simulink model "Scenario_1"  (R2020b)
settings: Solver=ode1  StartTime=0.0  StopTime=10  FixedStep=Ts  RelTol=1e-3
InitFcn:
  | Scenario_1_parameters;
values from neighbouring files (symbols this model uses):
  c0 = c0_zeb    (= 6.57988e-09)    [Scenario_17_parameters.m]    (also in Scenario_1_parameters.m = 6.37282e-09; Scenario_2_parameters.m = 6.37282e-09; Scenario_3_parameters.m)
  c1 = c1_zeb    (= 9.15905e-09)    [Scenario_17_parameters.m]    (also in Scenario_1_parameters.m = 8.76156e-09; Scenario_2_parameters.m = 8.76156e-09; Scenario_3_parameters.m)
  fg = 50    [Scenario_17_parameters.m]    (also in Scenario_1_parameters.m; Scenario_2_parameters.m; Scenario_3_parameters.m)
  G1gen = 0.50    (= 0.5)    [Scenario_17_parameters.m]    (also in Scenario_1_parameters.m = 0.2; Scenario_2_parameters.m = 0.1245; Scenario_3_parameters.m = 0.45)
  G2gen = 0.30    (= 0.3)    [Scenario_1_parameters.m]    (also in Scenario_2_parameters.m; Scenario_3_parameters.m = 0.4)
  G3gen = 0.25    [Scenario_1_parameters.m]    (also in Scenario_2_parameters.m = 0.2; Scenario_3_parameters.m = 0.6)
  G5gen = 0.75    [Scenario_17_parameters.m]    (also in Scenario_1_parameters.m = 0.22; Scenario_2_parameters.m = 0.2; Scenario_3_parameters.m = 0.7)
  G6gen = 0.90    (= 0.9)    [Scenario_17_parameters.m]    (also in Scenario_1_parameters.m = 0.41; Scenario_2_parameters.m = 0.2078; Scenario_3_parameters.m = 0.95)
  G7gen = 0.60    (= 0.6)    [Scenario_17_parameters.m]    (also in Scenario_1_parameters.m = 0.52; Scenario_2_parameters.m = 0.518; Scenario_3_parameters.m = 0.5)
  Ihvpk = Ihv*sqrt(2)    [Scenario_17_parameters.m]    (also in Scenario_1_parameters.m; Scenario_2_parameters.m; Scenario_3_parameters.m)
  l0 = l0_zeb    (= 0.00368)    [Scenario_17_parameters.m]    (also in Scenario_1_parameters.m = 0.00373; Scenario_2_parameters.m = 0.00373; Scenario_3_parameters.m)
  l1 = l1_zeb    (= 0.00128)    [Scenario_17_parameters.m]    (also in Scenario_1_parameters.m = 0.00133; Scenario_2_parameters.m = 0.00133; Scenario_3_parameters.m)
  L3dem = 0.30    (= 0.3)    [Scenario_17_parameters.m]    (also in Scenario_1_parameters.m = 0.1; Scenario_2_parameters.m = 0.1; Scenario_3_parameters.m = 0.2)
  L4dem = 0.30    (= 0.3)    [Scenario_1_parameters.m]    (also in Scenario_2_parameters.m)
  L5dem = 0.25    [Scenario_17_parameters.m]    (also in Scenario_1_parameters.m = 0.35; Scenario_2_parameters.m = 0.35)
  L6dem = 0.15    [Scenario_1_parameters.m]    (also in Scenario_2_parameters.m; Scenario_3_parameters.m = 0.1)
  L7dem = 0.10    (= 0.1)    [Scenario_1_parameters.m]    (also in Scenario_2_parameters.m; Scenario_3_parameters.m = 0.15)
  Pr = Sr*PF    (= 1900000000)    [Scenario_17_parameters.m]    (also in Scenario_1_parameters.m = 550050000; Scenario_2_parameters.m = 550050000; Scenario_3_parameters.m = 11640000000)
  Qr = sqrt(Sr^2 - Pr^2)    [Scenario_17_parameters.m]    (also in Scenario_1_parameters.m; Scenario_2_parameters.m; Scenario_3_parameters.m)
  r0 = r0_zeb    (= 0.39362)    [Scenario_17_parameters.m]    (also in Scenario_1_parameters.m = 0.44587; Scenario_2_parameters.m = 0.44587; Scenario_3_parameters.m)
  r1 = r1_zeb    (= 0.06862)    [Scenario_17_parameters.m]    (also in Scenario_1_parameters.m = 0.12087; Scenario_2_parameters.m = 0.12087; Scenario_3_parameters.m)
  Rtpu = Xtpu/40    (= 0.0025)    [Scenario_17_parameters.m]    (also in Scenario_1_parameters.m = 0.00375; Scenario_2_parameters.m = 0.00375; Scenario_3_parameters.m = 0.00375)
  S1non = 700e6    (= 700000000)    [Scenario_17_parameters.m]    (also in Scenario_1_parameters.m = 400000000; Scenario_2_parameters.m = 400000000; Scenario_3_parameters.m = 1000000000)
  S2non = 300e6    (= 300000000)    [Scenario_1_parameters.m]    (also in Scenario_2_parameters.m; Scenario_3_parameters.m = 3000000000)
  S3non = 200e6    (= 200000000)    [Scenario_1_parameters.m]    (also in Scenario_2_parameters.m; Scenario_3_parameters.m = 1000000000)
  S5non = 400e6    (= 400000000)    [Scenario_17_parameters.m]    (also in Scenario_1_parameters.m = 500000000; Scenario_2_parameters.m = 500000000; Scenario_3_parameters.m = 2000000000)
  S6non = 150e6    (= 150000000)    [Scenario_17_parameters.m]    (also in Scenario_1_parameters.m = 400000000; Scenario_2_parameters.m = 400000000; Scenario_3_parameters.m = 3000000000)
  S7non = 1000e6    (= 1000000000)    [Scenario_17_parameters.m]    (also in Scenario_1_parameters.m = 200000000; Scenario_2_parameters.m = 200000000; Scenario_3_parameters.m = 4000000000)
  tonvsc = 0.01    [Scenario_17_parameters.m]    (also in Scenario_1_parameters.m = 0.02; Scenario_2_parameters.m; Scenario_3_parameters.m = 0.05)
  Ts = 100e-6    (= 0.0001)    [Scenario_17_parameters.m]    (also in Scenario_1_parameters.m; Scenario_2_parameters.m; Scenario_3_parameters.m = 5e-05)
  Vhv = 220e3    (= 220000)    [Scenario_17_parameters.m]    (also in Scenario_1_parameters.m; Scenario_2_parameters.m; Scenario_3_parameters.m)
  Vmv = 22e3    (= 22000)    [Scenario_17_parameters.m]    (also in Scenario_1_parameters.m; Scenario_2_parameters.m; Scenario_3_parameters.m)
  wc1 = wsw1/10    (= 848.230016469)    [Scenario_17_parameters.m]    (also in Scenario_1_parameters.m; Scenario_2_parameters.m; Scenario_3_parameters.m)
  wdc1 = wc1/10    (= 84.8230016469)    [Scenario_17_parameters.m]    (also in Scenario_1_parameters.m; Scenario_2_parameters.m; Scenario_3_parameters.m)
  wpq1 = wc1/10    (= 84.8230016469)    [Scenario_17_parameters.m]    (also in Scenario_1_parameters.m; Scenario_2_parameters.m; Scenario_3_parameters.m)
  wsw1 = ksw1*2*pi*fg    (= 8482.30016469)    [Scenario_17_parameters.m]    (also in Scenario_1_parameters.m; Scenario_2_parameters.m; Scenario_3_parameters.m)
  Xtpu = 0.10    (= 0.1)    [Scenario_17_parameters.m]    (also in Scenario_1_parameters.m = 0.15; Scenario_2_parameters.m = 0.15; Scenario_3_parameters.m = 0.15)
undefined symbols (not defined in the file or in its folder): D11, Delta, Kf, r, theta0
libraries: powerlib x206, simulink_extras x140, powerlib_meascontrol x82, pid_lib x48, eeGeneralControl x32, simulink x28, eeTransforms x24, spsFirstOrderFilterLib x16, eePwmGeneratorTwoLevel x4
(part 5 of 16)

== system Scenario_1/G7/Exciter System/SEXS ==
  note: The controller parameters provided by ENTSO-E
      | define different names for the parameters:
      |
      | ENTSO-E = IEEE Std 421.5-2005
      | Ta = Tc
      | Tb = Tb
      | K = Ka
      | Te = Ta
      | Emax = Vrmax
      | Emin = Vrmin
  note: The exciter model provided by ENTSO-E most similar to the IEEE is the Type AC4A excitation system model
  Vref : Inport
  Vc : Inport  Port=2
  Vs : Inport  Port=3
  1st ord transfer fcn windup limiter : Subsystem  mask{Gain=K, tau=Te, Vmax=Emax, Vmin=Emin, y0=Vf0}
      mask prompts: tau "Time constant"; y0 "Initial output"
  Constant : Constant  Value=Vf0/K
  Saturation : Saturate  Commented=through  UpperLimit=0.1  LowerLimit=-0.1
  Sum : Sum  Inputs=+-+
  Sum1 : Sum  Inputs=|++
  Transfer Fcn (with initial outputs)1 : simulink_extras/Additional Linear/Transfer Fcn (with initial outputs)  N=[Ta 1]  D=[Tb 1]  Y0=Vf0/K  U0=Vf0/K
  Efd : Outport
  wires:
  1st ord transfer fcn windup limiter/1(Out1) -> Efd/1
  Vs/1 -> Sum/3
  Vref/1 -> Sum/1
  Vc/1 -> Sum/2
  Transfer Fcn (with initial outputs)1/1 -> 1st ord transfer fcn windup limiter/1(In1)
  Saturation/1 -> Transfer Fcn (with initial outputs)1/1
  Sum/1 -> Sum1/1
  Sum1/1 -> Saturation/1
  Constant/1 -> Sum1/2

== system Scenario_1/G7/Exciter System/TR and LC_test ==
  note: Terminal voltage transducer and optional load compensation
  note: compensated
      | impedance
  note: Vt and It should be phasors (complex quantities)
  note: Fig 4.1 of IEEE Std 421.5-2005
  note: Rc and Xc should be negative values in case of voltage regulated after an impedance
  Vt : Inport
  It : Inport  Port=2
  Abs : Abs
  Abs1 : Abs
  Rc+jXc : Gain  Gain=abs(Rc+1i*Xc)
  Saturation : Saturate  UpperLimit=1.2  LowerLimit=0.8
  Sum : Sum  Inputs=|+-
  Transfer Fcn (with initial outputs) : simulink_extras/Additional Linear/Transfer Fcn (with initial outputs)  Commented=through  N=[1]  D=[Tr 1]  Y0=1  U0=1
  Vc : Outport
  wires:
  Saturation/1 -> Vc/1
  Vt/1 -> Abs/1
  Transfer Fcn (with initial outputs)/1 -> Saturation/1
  Rc+jXc/1 -> Sum/2
  Sum/1 -> Transfer Fcn (with initial outputs)/1
  It/1 -> Abs1/1
  Abs/1 -> Sum/1
  Abs1/1 -> Rc+jXc/1

== system Scenario_1/G1/Exciter System/SEXS/1st ord transfer fcn windup limiter ==
  note: First order transfer function with windup limiter (non-saturated output)
  In1 : Inport
  Compare To Constant : simulink/Logic and Bit Operations/Compare To Constant  relop=<=  const=Vmax  OutDataTypeStr=boolean
  Compare To Constant1 : simulink/Logic and Bit Operations/Compare To Constant  relop=>=  const=Vmin  OutDataTypeStr=boolean
  OR : Logic  Operator=OR  IconShape=distinctive  AllPortsSameDT=off  OutDataTypeStr=boolean
  Sample and Hold1 : powerlib_meascontrol/Additional Components/Sample and Hold  ic=0  Ts=0
      settings: SourceProductBaseCode=PS
  Saturation1 : Saturate  UpperLimit=Vmax  LowerLimit=Vmin
  Transfer Fcn (with initial outputs)2 : simulink_extras/Additional Linear/Transfer Fcn (with initial outputs)  N=[Gain]  D=[tau 1]  Y0=y0  U0=y0/Gain
  Out1 : Outport
  wires:
  Sample and Hold1/1 -> Transfer Fcn (with initial outputs)2/1
  Transfer Fcn (with initial outputs)2/1 -> Saturation1/1, Compare To Constant1/1, Compare To Constant/1
  In1/1 -> Sample and Hold1/1
  Compare To Constant/1 -> OR/1
  Compare To Constant1/1 -> OR/2
  OR/1 -> Sample and Hold1/2
  Saturation1/1 -> Out1/1

== system Scenario_1/G2/VSC/VSC Control/Control loops ==
  note: 1) Add Subsystem or Model blocks as valid variant choices.
      | 2) You cannot connect blocks at this level. At simulation, connectivity is automatically
      | determined, based on the active variant and port name matching.
  Pset : Inport
  Qset : Inport  Port=2
  vqd+- : Inport  Port=3
  iqd+- : Inport  Port=4
  freq : Inport  Port=5
  Block : Inport  Port=6
  Phasor I 1st : Subsystem  VariantControl=Phasor_I_1st
  Phasor I ref : Subsystem  VariantControl=Phasor_I_ref
  Phasor PQ 1st : Subsystem  VariantControl=Phasor_PQ
  "SW, EMT AVG, Phasor Quasi-EMT" : Subsystem  VariantControl=EMT_and_QEMT
  vqd+-ref : Outport
  iqd+-ref : Outport  Port=2
  m : Outport  Port=3

== system Scenario_1/G2/VSC/VSC Control/Measurements ==
  note: 1) Add Subsystem or Model blocks as valid variant choices.
      | 2) You cannot connect blocks at this level. At simulation, connectivity is automatically
      | determined, based on the active variant and port name matching.
  Vabc : Inport
  Iabc : Inport  Port=2
  EMT : Subsystem  VariantControl=EMT
  Phasor : Subsystem  VariantControl=Phasor
  vqd+- : Outport
  iqd+- : Outport  Port=2
  freq : Outport  Port=3
  theta : Outport  Port=4
  PQabc : Outport  Port=5

== system Scenario_1/G2/VSC/VSC Control/Modulation ==
  note: 1) Add Subsystem or Model blocks as valid variant choices.
      | 2) You cannot connect blocks at this level. At simulation, connectivity is automatically
      | determined, based on the active variant and port name matching.
  vqd+- : Inport
  vqd+-* : Inport  Port=2
  iqd+-* : Inport  Port=3
  theta : Inport  Port=4
  EMT AVG : Subsystem  VariantControl=EMT_AVG
  EMT Switching : Subsystem  VariantControl=EMT_SW
  Phasor I and Phasor PQ : Subsystem  VariantControl=Phasor_I_and_PQ
  Phasor Quasi-EMT : Subsystem  VariantControl=Phasor_QEMT
  Ref : Outport

== system Scenario_1/G2/VSC/VSC Model/EMT AVG ==
  Ref : Inport
  Controlled Voltage Source3 : powerlib/Electrical Sources/Controlled Voltage Source  Initialize=off  Source_Type=AC  Amplitude=Vhvpk  Phase=0  Frequency=fg  Measurements=None
  Controlled Voltage Source4 : powerlib/Electrical Sources/Controlled Voltage Source  Initialize=off  Source_Type=AC  Amplitude=Vhvpk  Phase=-2*pi/3  Frequency=fg  Measurements=None
  Controlled Voltage Source5 : powerlib/Electrical Sources/Controlled Voltage Source  Initialize=off  Source_Type=AC  Amplitude=Vhvpk  Phase=-4*pi/3  Frequency=fg  Measurements=None
  Demux1 : Demux  Outputs=3
  Ground : powerlib/Elements/Ground  LConnTagsString=a
  Ground4 : powerlib/Elements/Ground  LConnTagsString=a
  Ground5 : powerlib/Elements/Ground  LConnTagsString=a
  A : PMIOPort  Side=Left
  B : PMIOPort  Port=2  Side=Left
  C : PMIOPort  Port=3  Side=Left
  wires:
  Ref/1 -> Demux1/1
  Demux1/1 -> Controlled Voltage Source3/1
  Demux1/2 -> Controlled Voltage Source4/1
  Demux1/3 -> Controlled Voltage Source5/1
  connections:
  Controlled Voltage Source3/RConn1 -- A/RConn1
  Controlled Voltage Source4/RConn1 -- B/RConn1
  Controlled Voltage Source5/RConn1 -- C/RConn1
  Ground/LConn1 -- Controlled Voltage Source3/LConn1
  Ground4/LConn1 -- Controlled Voltage Source4/LConn1
  Ground5/LConn1 -- Controlled Voltage Source5/LConn1

== system Scenario_1/G2/VSC/VSC Model/EMT SW ==
  Ref : Inport
  DC Voltage Source : powerlib/Electrical Sources/DC Voltage Source  Amplitude=Vdc  Measurements=None
  Universal Bridge : powerlib/Power Electronics/Universal Bridge  Arms=3  SnubberResistance=1e6  SnubberCapacitance=inf  Device=IGBT / Diodes  Ron=1e-4  Lon=0  ForwardVoltages="[  0  0  ]"  ForwardVoltage=0  GTOparameters=[ 10e-6 , 20e-6 ]  IGBTparameters=[ 1e-6 , 2e-6 ]  Measurements=None  Measurements_2=None  converterType=Rectifier
  A : PMIOPort  Side=Left
  B : PMIOPort  Port=2  Side=Left
  C : PMIOPort  Port=3  Side=Left
  wires:
  Ref/1 -> Universal Bridge/1
  connections:
  Universal Bridge/LConn2 -- B/RConn1
  Universal Bridge/LConn1 -- A/RConn1
  Universal Bridge/LConn3 -- C/RConn1
  Universal Bridge/RConn1 -- DC Voltage Source/RConn1
  Universal Bridge/RConn2 -- DC Voltage Source/LConn1

== system Scenario_1/G2/VSC/VSC Model/Phasor ==
  Ref : Inport
  Controlled Current Source : powerlib/Electrical Sources/Controlled Current Source  Initialize=off  Source_Type=AC  Amplitude=0  Phase=0  Frequency=0  Measurements=None
  Controlled Current Source1 : powerlib/Electrical Sources/Controlled Current Source  Initialize=off  Source_Type=AC  Amplitude=0  Phase=0  Frequency=0  Measurements=None
  Controlled Current Source2 : powerlib/Electrical Sources/Controlled Current Source  Initialize=off  Source_Type=AC  Amplitude=0  Phase=0  Frequency=0  Measurements=None
  Demux1 : Demux  Outputs=3
  Ground{1..3,5} (4 alike) : powerlib/Elements/Ground  LConnTagsString=a
  Three-Phase Series RLC Branch : powerlib/Elements/Three-Phase Series RLC Branch  LConnTagsString=A|B|C  RConnTagsString=A|B|C  BranchType=R  Resistance=1e7  Inductance=1e-3  Capacitance=1e-6  Measurements=None
  A : PMIOPort  Side=Left
  B : PMIOPort  Port=2  Side=Left
  C : PMIOPort  Port=3  Side=Left
  wires:
  [c] -> Controlled Current Source2/1
  [b] -> Controlled Current Source1/1
  [a] -> Controlled Current Source/1
  Demux1/3 -> [c]
  Demux1/2 -> [b]
  Demux1/1 -> [a]
  Ref/1 -> Demux1/1
  connections:
  Controlled Current Source/RConn1 -- Ground1/LConn1
  Controlled Current Source1/RConn1 -- Ground2/LConn1
  Controlled Current Source2/RConn1 -- Ground3/LConn1
  A/RConn1 -- Controlled Current Source/LConn1 -- Three-Phase Series RLC Branch/LConn1
  C/RConn1 -- Controlled Current Source2/LConn1 -- Three-Phase Series RLC Branch/LConn3
  Ground5/LConn1 -- Three-Phase Series RLC Branch/RConn2 -- Three-Phase Series RLC Branch/RConn1 -- Three-Phase Series RLC Branch/RConn3
  Controlled Current Source1/LConn1 -- Three-Phase Series RLC Branch/LConn2 -- B/RConn1

== system Scenario_1/G3/VSC/VSC Control/Control loops ==
  note: 1) Add Subsystem or Model blocks as valid variant choices.
      | 2) You cannot connect blocks at this level. At simulation, connectivity is automatically
      | determined, based on the active variant and port name matching.
  Pset : Inport
  Qset : Inport  Port=2
  vqd+- : Inport  Port=3
  iqd+- : Inport  Port=4
  freq : Inport  Port=5
  Block : Inport  Port=6
  Phasor I 1st : Subsystem  VariantControl=Phasor_I_1st
  Phasor I ref : Subsystem  VariantControl=Phasor_I_ref
  Phasor PQ 1st : Subsystem  VariantControl=Phasor_PQ
  "SW, EMT AVG, Phasor Quasi-EMT" : Subsystem  VariantControl=EMT_and_QEMT
  vqd+-ref : Outport
  iqd+-ref : Outport  Port=2
  m : Outport  Port=3

== system Scenario_1/G3/VSC/VSC Control/Measurements ==
  note: 1) Add Subsystem or Model blocks as valid variant choices.
      | 2) You cannot connect blocks at this level. At simulation, connectivity is automatically
      | determined, based on the active variant and port name matching.
  Vabc : Inport
  Iabc : Inport  Port=2
  EMT : Subsystem  VariantControl=EMT
  Phasor : Subsystem  VariantControl=Phasor
  vqd+- : Outport
  iqd+- : Outport  Port=2
  freq : Outport  Port=3
  theta : Outport  Port=4
  PQabc : Outport  Port=5

== system Scenario_1/G3/VSC/VSC Control/Modulation ==
  note: 1) Add Subsystem or Model blocks as valid variant choices.
      | 2) You cannot connect blocks at this level. At simulation, connectivity is automatically
      | determined, based on the active variant and port name matching.
  vqd+- : Inport
  vqd+-* : Inport  Port=2
  iqd+-* : Inport  Port=3
  theta : Inport  Port=4
  EMT AVG : Subsystem  VariantControl=EMT_AVG
  EMT Switching : Subsystem  VariantControl=EMT_SW
  Phasor I and Phasor PQ : Subsystem  VariantControl=Phasor_I_and_PQ
  Phasor Quasi-EMT : Subsystem  VariantControl=Phasor_QEMT
  Ref : Outport

== system Scenario_1/G3/VSC/VSC Model/EMT AVG ==
  Ref : Inport
  Controlled Voltage Source3 : powerlib/Electrical Sources/Controlled Voltage Source  Initialize=off  Source_Type=AC  Amplitude=Vhvpk  Phase=0  Frequency=fg  Measurements=None
  Controlled Voltage Source4 : powerlib/Electrical Sources/Controlled Voltage Source  Initialize=off  Source_Type=AC  Amplitude=Vhvpk  Phase=-2*pi/3  Frequency=fg  Measurements=None
  Controlled Voltage Source5 : powerlib/Electrical Sources/Controlled Voltage Source  Initialize=off  Source_Type=AC  Amplitude=Vhvpk  Phase=-4*pi/3  Frequency=fg  Measurements=None
  Demux1 : Demux  Outputs=3
  Ground : powerlib/Elements/Ground  LConnTagsString=a
  Ground4 : powerlib/Elements/Ground  LConnTagsString=a
  Ground5 : powerlib/Elements/Ground  LConnTagsString=a
  A : PMIOPort  Side=Left
  B : PMIOPort  Port=2  Side=Left
  C : PMIOPort  Port=3  Side=Left
  wires:
  Ref/1 -> Demux1/1
  Demux1/1 -> Controlled Voltage Source3/1
  Demux1/2 -> Controlled Voltage Source4/1
  Demux1/3 -> Controlled Voltage Source5/1
  connections:
  Controlled Voltage Source3/RConn1 -- A/RConn1
  Controlled Voltage Source4/RConn1 -- B/RConn1
  Controlled Voltage Source5/RConn1 -- C/RConn1
  Ground/LConn1 -- Controlled Voltage Source3/LConn1
  Ground4/LConn1 -- Controlled Voltage Source4/LConn1
  Ground5/LConn1 -- Controlled Voltage Source5/LConn1

== system Scenario_1/G3/VSC/VSC Model/EMT SW ==
  Ref : Inport
  DC Voltage Source : powerlib/Electrical Sources/DC Voltage Source  Amplitude=Vdc  Measurements=None
  Universal Bridge : powerlib/Power Electronics/Universal Bridge  Arms=3  SnubberResistance=1e6  SnubberCapacitance=inf  Device=IGBT / Diodes  Ron=1e-4  Lon=0  ForwardVoltages="[  0  0  ]"  ForwardVoltage=0  GTOparameters=[ 10e-6 , 20e-6 ]  IGBTparameters=[ 1e-6 , 2e-6 ]  Measurements=None  Measurements_2=None  converterType=Rectifier
  A : PMIOPort  Side=Left
  B : PMIOPort  Port=2  Side=Left
  C : PMIOPort  Port=3  Side=Left
  wires:
  Ref/1 -> Universal Bridge/1
  connections:
  Universal Bridge/LConn2 -- B/RConn1
  Universal Bridge/LConn1 -- A/RConn1
  Universal Bridge/LConn3 -- C/RConn1
  Universal Bridge/RConn1 -- DC Voltage Source/RConn1
  Universal Bridge/RConn2 -- DC Voltage Source/LConn1

== system Scenario_1/G3/VSC/VSC Model/Phasor ==
  Ref : Inport
  Controlled Current Source : powerlib/Electrical Sources/Controlled Current Source  Initialize=off  Source_Type=AC  Amplitude=0  Phase=0  Frequency=0  Measurements=None
  Controlled Current Source1 : powerlib/Electrical Sources/Controlled Current Source  Initialize=off  Source_Type=AC  Amplitude=0  Phase=0  Frequency=0  Measurements=None
  Controlled Current Source2 : powerlib/Electrical Sources/Controlled Current Source  Initialize=off  Source_Type=AC  Amplitude=0  Phase=0  Frequency=0  Measurements=None
  Demux1 : Demux  Outputs=3
  Ground{1..3,5} (4 alike) : powerlib/Elements/Ground  LConnTagsString=a
  Three-Phase Series RLC Branch : powerlib/Elements/Three-Phase Series RLC Branch  LConnTagsString=A|B|C  RConnTagsString=A|B|C  BranchType=R  Resistance=1e7  Inductance=1e-3  Capacitance=1e-6  Measurements=None
  A : PMIOPort  Side=Left
  B : PMIOPort  Port=2  Side=Left
  C : PMIOPort  Port=3  Side=Left
  wires:
  [c] -> Controlled Current Source2/1
  [b] -> Controlled Current Source1/1
  [a] -> Controlled Current Source/1
  Demux1/3 -> [c]
  Demux1/2 -> [b]
  Demux1/1 -> [a]
  Ref/1 -> Demux1/1
  connections:
  Controlled Current Source/RConn1 -- Ground1/LConn1
  Controlled Current Source1/RConn1 -- Ground2/LConn1
  Controlled Current Source2/RConn1 -- Ground3/LConn1
  A/RConn1 -- Controlled Current Source/LConn1 -- Three-Phase Series RLC Branch/LConn1
  C/RConn1 -- Controlled Current Source2/LConn1 -- Three-Phase Series RLC Branch/LConn3
  Ground5/LConn1 -- Three-Phase Series RLC Branch/RConn2 -- Three-Phase Series RLC Branch/RConn1 -- Three-Phase Series RLC Branch/RConn3
  Controlled Current Source1/LConn1 -- Three-Phase Series RLC Branch/LConn2 -- B/RConn1

== system Scenario_1/G5/VSC/VSC Control/Control loops ==
  note: 1) Add Subsystem or Model blocks as valid variant choices.
      | 2) You cannot connect blocks at this level. At simulation, connectivity is automatically
      | determined, based on the active variant and port name matching.
  Pset : Inport
  Qset : Inport  Port=2
  vqd+- : Inport  Port=3
  iqd+- : Inport  Port=4
  freq : Inport  Port=5
  Block : Inport  Port=6
  Phasor I 1st : Subsystem  VariantControl=Phasor_I_1st
  Phasor I ref : Subsystem  VariantControl=Phasor_I_ref
  Phasor PQ 1st : Subsystem  VariantControl=Phasor_PQ
  "SW, EMT AVG, Phasor Quasi-EMT" : Subsystem  VariantControl=EMT_and_QEMT
  vqd+-ref : Outport
  iqd+-ref : Outport  Port=2
  m : Outport  Port=3

== system Scenario_1/G5/VSC/VSC Control/Measurements ==
  note: 1) Add Subsystem or Model blocks as valid variant choices.
      | 2) You cannot connect blocks at this level. At simulation, connectivity is automatically
      | determined, based on the active variant and port name matching.
  Vabc : Inport
  Iabc : Inport  Port=2
  EMT : Subsystem  VariantControl=EMT
  Phasor : Subsystem  VariantControl=Phasor
  vqd+- : Outport
  iqd+- : Outport  Port=2
  freq : Outport  Port=3
  theta : Outport  Port=4
  PQabc : Outport  Port=5

== system Scenario_1/G5/VSC/VSC Control/Modulation ==
  note: 1) Add Subsystem or Model blocks as valid variant choices.
      | 2) You cannot connect blocks at this level. At simulation, connectivity is automatically
      | determined, based on the active variant and port name matching.
  vqd+- : Inport
  vqd+-* : Inport  Port=2
  iqd+-* : Inport  Port=3
  theta : Inport  Port=4
  EMT AVG : Subsystem  VariantControl=EMT_AVG
  EMT Switching : Subsystem  VariantControl=EMT_SW
  Phasor I and Phasor PQ : Subsystem  VariantControl=Phasor_I_and_PQ
  Phasor Quasi-EMT : Subsystem  VariantControl=Phasor_QEMT
  Ref : Outport

== system Scenario_1/G5/VSC/VSC Model/EMT AVG ==
  Ref : Inport
  Controlled Voltage Source3 : powerlib/Electrical Sources/Controlled Voltage Source  Initialize=off  Source_Type=AC  Amplitude=Vhvpk  Phase=0  Frequency=fg  Measurements=None
  Controlled Voltage Source4 : powerlib/Electrical Sources/Controlled Voltage Source  Initialize=off  Source_Type=AC  Amplitude=Vhvpk  Phase=-2*pi/3  Frequency=fg  Measurements=None
  Controlled Voltage Source5 : powerlib/Electrical Sources/Controlled Voltage Source  Initialize=off  Source_Type=AC  Amplitude=Vhvpk  Phase=-4*pi/3  Frequency=fg  Measurements=None
  Demux1 : Demux  Outputs=3
  Ground : powerlib/Elements/Ground  LConnTagsString=a
  Ground4 : powerlib/Elements/Ground  LConnTagsString=a
  Ground5 : powerlib/Elements/Ground  LConnTagsString=a
  A : PMIOPort  Side=Left
  B : PMIOPort  Port=2  Side=Left
  C : PMIOPort  Port=3  Side=Left
  wires:
  Ref/1 -> Demux1/1
  Demux1/1 -> Controlled Voltage Source3/1
  Demux1/2 -> Controlled Voltage Source4/1
  Demux1/3 -> Controlled Voltage Source5/1
  connections:
  Controlled Voltage Source3/RConn1 -- A/RConn1
  Controlled Voltage Source4/RConn1 -- B/RConn1
  Controlled Voltage Source5/RConn1 -- C/RConn1
  Ground/LConn1 -- Controlled Voltage Source3/LConn1
  Ground4/LConn1 -- Controlled Voltage Source4/LConn1
  Ground5/LConn1 -- Controlled Voltage Source5/LConn1

== system Scenario_1/G5/VSC/VSC Model/EMT SW ==
  Ref : Inport
  DC Voltage Source : powerlib/Electrical Sources/DC Voltage Source  Amplitude=Vdc  Measurements=None
  Universal Bridge : powerlib/Power Electronics/Universal Bridge  Arms=3  SnubberResistance=1e6  SnubberCapacitance=inf  Device=IGBT / Diodes  Ron=1e-4  Lon=0  ForwardVoltages="[  0  0  ]"  ForwardVoltage=0  GTOparameters=[ 10e-6 , 20e-6 ]  IGBTparameters=[ 1e-6 , 2e-6 ]  Measurements=None  Measurements_2=None  converterType=Rectifier
  A : PMIOPort  Side=Left
  B : PMIOPort  Port=2  Side=Left
  C : PMIOPort  Port=3  Side=Left
  wires:
  Ref/1 -> Universal Bridge/1
  connections:
  Universal Bridge/LConn2 -- B/RConn1
  Universal Bridge/LConn1 -- A/RConn1
  Universal Bridge/LConn3 -- C/RConn1
  Universal Bridge/RConn1 -- DC Voltage Source/RConn1
  Universal Bridge/RConn2 -- DC Voltage Source/LConn1

== system Scenario_1/G5/VSC/VSC Model/Phasor ==
  Ref : Inport
  Controlled Current Source : powerlib/Electrical Sources/Controlled Current Source  Initialize=off  Source_Type=AC  Amplitude=0  Phase=0  Frequency=0  Measurements=None
  Controlled Current Source1 : powerlib/Electrical Sources/Controlled Current Source  Initialize=off  Source_Type=AC  Amplitude=0  Phase=0  Frequency=0  Measurements=None
  Controlled Current Source2 : powerlib/Electrical Sources/Controlled Current Source  Initialize=off  Source_Type=AC  Amplitude=0  Phase=0  Frequency=0  Measurements=None
  Demux1 : Demux  Outputs=3
  Ground{1..3,5} (4 alike) : powerlib/Elements/Ground  LConnTagsString=a
  Three-Phase Series RLC Branch : powerlib/Elements/Three-Phase Series RLC Branch  LConnTagsString=A|B|C  RConnTagsString=A|B|C  BranchType=R  Resistance=1e7  Inductance=1e-3  Capacitance=1e-6  Measurements=None
  A : PMIOPort  Side=Left
  B : PMIOPort  Port=2  Side=Left
  C : PMIOPort  Port=3  Side=Left
  wires:
  [c] -> Controlled Current Source2/1
  [b] -> Controlled Current Source1/1
  [a] -> Controlled Current Source/1
  Demux1/3 -> [c]
  Demux1/2 -> [b]
  Demux1/1 -> [a]
  Ref/1 -> Demux1/1
  connections:
  Controlled Current Source/RConn1 -- Ground1/LConn1
  Controlled Current Source1/RConn1 -- Ground2/LConn1
  Controlled Current Source2/RConn1 -- Ground3/LConn1
  A/RConn1 -- Controlled Current Source/LConn1 -- Three-Phase Series RLC Branch/LConn1
  C/RConn1 -- Controlled Current Source2/LConn1 -- Three-Phase Series RLC Branch/LConn3
  Ground5/LConn1 -- Three-Phase Series RLC Branch/RConn2 -- Three-Phase Series RLC Branch/RConn1 -- Three-Phase Series RLC Branch/RConn3
  Controlled Current Source1/LConn1 -- Three-Phase Series RLC Branch/LConn2 -- B/RConn1

== system Scenario_1/G6/VSC/VSC Control/Control loops ==
  note: 1) Add Subsystem or Model blocks as valid variant choices.
      | 2) You cannot connect blocks at this level. At simulation, connectivity is automatically
      | determined, based on the active variant and port name matching.
  Pset : Inport
  Qset : Inport  Port=2
  vqd+- : Inport  Port=3
  iqd+- : Inport  Port=4
  freq : Inport  Port=5
  Block : Inport  Port=6
  Phasor I 1st : Subsystem  VariantControl=Phasor_I_1st
  Phasor I ref : Subsystem  VariantControl=Phasor_I_ref
  Phasor PQ 1st : Subsystem  VariantControl=Phasor_PQ
  "SW, EMT AVG, Phasor Quasi-EMT" : Subsystem  VariantControl=EMT_and_QEMT
  vqd+-ref : Outport
  iqd+-ref : Outport  Port=2
  m : Outport  Port=3

== system Scenario_1/G6/VSC/VSC Control/Measurements ==
  note: 1) Add Subsystem or Model blocks as valid variant choices.
      | 2) You cannot connect blocks at this level. At simulation, connectivity is automatically
      | determined, based on the active variant and port name matching.
  Vabc : Inport
  Iabc : Inport  Port=2
  EMT : Subsystem  VariantControl=EMT
  Phasor : Subsystem  VariantControl=Phasor
  vqd+- : Outport
  iqd+- : Outport  Port=2
  freq : Outport  Port=3
  theta : Outport  Port=4
  PQabc : Outport  Port=5

== system Scenario_1/G6/VSC/VSC Control/Modulation ==
  note: 1) Add Subsystem or Model blocks as valid variant choices.
      | 2) You cannot connect blocks at this level. At simulation, connectivity is automatically
      | determined, based on the active variant and port name matching.
  vqd+- : Inport
  vqd+-* : Inport  Port=2
  iqd+-* : Inport  Port=3
  theta : Inport  Port=4
  EMT AVG : Subsystem  VariantControl=EMT_AVG
  EMT Switching : Subsystem  VariantControl=EMT_SW
  Phasor I and Phasor PQ : Subsystem  VariantControl=Phasor_I_and_PQ
  Phasor Quasi-EMT : Subsystem  VariantControl=Phasor_QEMT
  Ref : Outport

== system Scenario_1/G6/VSC/VSC Model/EMT AVG ==
  Ref : Inport
  Controlled Voltage Source3 : powerlib/Electrical Sources/Controlled Voltage Source  Initialize=off  Source_Type=AC  Amplitude=Vhvpk  Phase=0  Frequency=fg  Measurements=None
  Controlled Voltage Source4 : powerlib/Electrical Sources/Controlled Voltage Source  Initialize=off  Source_Type=AC  Amplitude=Vhvpk  Phase=-2*pi/3  Frequency=fg  Measurements=None
  Controlled Voltage Source5 : powerlib/Electrical Sources/Controlled Voltage Source  Initialize=off  Source_Type=AC  Amplitude=Vhvpk  Phase=-4*pi/3  Frequency=fg  Measurements=None
  Demux1 : Demux  Outputs=3
  Ground : powerlib/Elements/Ground  LConnTagsString=a
  Ground4 : powerlib/Elements/Ground  LConnTagsString=a
  Ground5 : powerlib/Elements/Ground  LConnTagsString=a
  A : PMIOPort  Side=Left
  B : PMIOPort  Port=2  Side=Left
  C : PMIOPort  Port=3  Side=Left
  wires:
  Ref/1 -> Demux1/1
  Demux1/1 -> Controlled Voltage Source3/1
  Demux1/2 -> Controlled Voltage Source4/1
  Demux1/3 -> Controlled Voltage Source5/1
  connections:
  Controlled Voltage Source3/RConn1 -- A/RConn1
  Controlled Voltage Source4/RConn1 -- B/RConn1
  Controlled Voltage Source5/RConn1 -- C/RConn1
  Ground/LConn1 -- Controlled Voltage Source3/LConn1
  Ground4/LConn1 -- Controlled Voltage Source4/LConn1
  Ground5/LConn1 -- Controlled Voltage Source5/LConn1

== system Scenario_1/G6/VSC/VSC Model/EMT SW ==
  Ref : Inport
  DC Voltage Source : powerlib/Electrical Sources/DC Voltage Source  Amplitude=Vdc  Measurements=None
  Universal Bridge : powerlib/Power Electronics/Universal Bridge  Arms=3  SnubberResistance=1e6  SnubberCapacitance=inf  Device=IGBT / Diodes  Ron=1e-4  Lon=0  ForwardVoltages="[  0  0  ]"  ForwardVoltage=0  GTOparameters=[ 10e-6 , 20e-6 ]  IGBTparameters=[ 1e-6 , 2e-6 ]  Measurements=None  Measurements_2=None  converterType=Rectifier
  A : PMIOPort  Side=Left
  B : PMIOPort  Port=2  Side=Left
  C : PMIOPort  Port=3  Side=Left
  wires:
  Ref/1 -> Universal Bridge/1
  connections:
  Universal Bridge/LConn2 -- B/RConn1
  Universal Bridge/LConn1 -- A/RConn1
  Universal Bridge/LConn3 -- C/RConn1
  Universal Bridge/RConn1 -- DC Voltage Source/RConn1
  Universal Bridge/RConn2 -- DC Voltage Source/LConn1

== system Scenario_1/G6/VSC/VSC Model/Phasor ==
  Ref : Inport
  Controlled Current Source : powerlib/Electrical Sources/Controlled Current Source  Initialize=off  Source_Type=AC  Amplitude=0  Phase=0  Frequency=0  Measurements=None
  Controlled Current Source1 : powerlib/Electrical Sources/Controlled Current Source  Initialize=off  Source_Type=AC  Amplitude=0  Phase=0  Frequency=0  Measurements=None
  Controlled Current Source2 : powerlib/Electrical Sources/Controlled Current Source  Initialize=off  Source_Type=AC  Amplitude=0  Phase=0  Frequency=0  Measurements=None
  Demux1 : Demux  Outputs=3
  Ground{1..3,5} (4 alike) : powerlib/Elements/Ground  LConnTagsString=a
  Three-Phase Series RLC Branch : powerlib/Elements/Three-Phase Series RLC Branch  LConnTagsString=A|B|C  RConnTagsString=A|B|C  BranchType=R  Resistance=1e7  Inductance=1e-3  Capacitance=1e-6  Measurements=None
  A : PMIOPort  Side=Left
  B : PMIOPort  Port=2  Side=Left
  C : PMIOPort  Port=3  Side=Left
  wires:
  [c] -> Controlled Current Source2/1
  [b] -> Controlled Current Source1/1
  [a] -> Controlled Current Source/1
  Demux1/3 -> [c]
  Demux1/2 -> [b]
  Demux1/1 -> [a]
  Ref/1 -> Demux1/1
  connections:
  Controlled Current Source/RConn1 -- Ground1/LConn1
  Controlled Current Source1/RConn1 -- Ground2/LConn1
  Controlled Current Source2/RConn1 -- Ground3/LConn1
  A/RConn1 -- Controlled Current Source/LConn1 -- Three-Phase Series RLC Branch/LConn1
  C/RConn1 -- Controlled Current Source2/LConn1 -- Three-Phase Series RLC Branch/LConn3
  Ground5/LConn1 -- Three-Phase Series RLC Branch/RConn2 -- Three-Phase Series RLC Branch/RConn1 -- Three-Phase Series RLC Branch/RConn3
  Controlled Current Source1/LConn1 -- Three-Phase Series RLC Branch/LConn2 -- B/RConn1

== system Scenario_1/G7/Exciter System/SEXS/1st ord transfer fcn windup limiter ==
  note: First order transfer function with windup limiter (non-saturated output)
  In1 : Inport
  Compare To Constant : simulink/Logic and Bit Operations/Compare To Constant  relop=<=  const=Vmax  OutDataTypeStr=boolean
  Compare To Constant1 : simulink/Logic and Bit Operations/Compare To Constant  relop=>=  const=Vmin  OutDataTypeStr=boolean
  OR : Logic  Operator=OR  IconShape=distinctive  AllPortsSameDT=off  OutDataTypeStr=boolean
  Sample and Hold1 : powerlib_meascontrol/Additional Components/Sample and Hold  ic=0  Ts=0
      settings: SourceProductBaseCode=PS
  Saturation1 : Saturate  UpperLimit=Vmax  LowerLimit=Vmin
  Transfer Fcn (with initial outputs)2 : simulink_extras/Additional Linear/Transfer Fcn (with initial outputs)  N=[Gain]  D=[tau 1]  Y0=y0  U0=y0/Gain
  Out1 : Outport
  wires:
  Sample and Hold1/1 -> Transfer Fcn (with initial outputs)2/1
  Transfer Fcn (with initial outputs)2/1 -> Saturation1/1, Compare To Constant1/1, Compare To Constant/1
  In1/1 -> Sample and Hold1/1
  Compare To Constant/1 -> OR/1
  Compare To Constant1/1 -> OR/2
  OR/1 -> Sample and Hold1/2
  Saturation1/1 -> Out1/1

== system Scenario_1/G2/VSC/VSC Control/Control loops/Phasor I 1st ==
  Pset : Inport
  Qset : Inport  Port=2
  vqd+- : Inport  Port=3
  iqd+- : Inport  Port=4
  freq : Inport  Port=5
  Block : Inport  Port=6
  Inner-loop : Subsystem
  Mux : Mux
  Outer-loop : Subsystem
      settings: PortSchema="{\"entries\":[{\"content\":{\"sides\":[{\"content\":{\"connectorIds\":[\"In1\",\"In2\",\"In3\",\"In4\",\"In5\"]},\"type\":\"ConnectorPlacement.EquallySpacedRectSide\",\"uuid\":\"9a334ab0-c6a2-41fb-a6ec-750715335523\"},{\"content\":{\"connectorIds\":[\"Out1\",\"Out2\",\"Out3\",\"Out4\",\"Out5\"],\"side\":\"RIGHT\"},\"type\":\"ConnectorPlacement.EquallySpacedRectSide\",\"uuid\":\"d3309230-0110-441f-b944-3d5d4312a42e\"},{\"content\":{\"connectorIds\":[\"In6\"],\"side\":\"TOP\"},\"type\":\"ConnectorPlacement.EquallySpacedRectSide\",\"uuid\":\"012603a1-4678-4ae1-91f6-3e17a1c8130b\"}]},\"type\":\"ConnectorPlacement.EquallySpacedConnector\",\"uuid\":\"299866d5-057c-44fe-b725-733ff7b8fc12\"}],\"packageUris\":[\"http://schema.mathworks.com/mf0/Connector/19700101\"],\"version\":\"1.0\"}"
  iqd+-ref : Outport
  m : Outport  Port=2
  wires:
  Outer-loop/4(id-*) -> Inner-loop/4(id-*)
  Outer-loop/3(iq-*) -> Inner-loop/3(iq-*)
  Outer-loop/2(id+*) -> Inner-loop/2(id+*)
  Outer-loop/1(iq+*) -> Inner-loop/1(iq+*)
  Block/1 -> Outer-loop/6(Blk)
  vqd+-/1 -> Outer-loop/3(vqd+-)
  freq/1 -> Outer-loop/5(freq)
  iqd+-/1 -> Outer-loop/4(iqd+-)
  Inner-loop/2(id+ref) -> Mux/2
  Pset/1 -> Outer-loop/1(Pset)
  Outer-loop/5(m) -> m/1
  Qset/1 -> Outer-loop/2(Qset)
  Mux/1 -> iqd+-ref/1
  Inner-loop/3(iq-ref) -> Mux/3
  Inner-loop/1(iq+ref) -> Mux/1
  Inner-loop/4(id-ref) -> Mux/4

== system Scenario_1/G2/VSC/VSC Control/Control loops/Phasor I ref ==
  Pset : Inport
  Qset : Inport  Port=2
  vqd+- : Inport  Port=3
  iqd+- : Inport  Port=4
  freq : Inport  Port=5
  Block : Inport  Port=6
  Mux : Mux
  Outer-loop : Subsystem
      settings: PortSchema="{\"entries\":[{\"content\":{\"sides\":[{\"content\":{\"connectorIds\":[\"In1\",\"In2\",\"In3\",\"In4\",\"In5\"]},\"type\":\"ConnectorPlacement.EquallySpacedRectSide\",\"uuid\":\"9a334ab0-c6a2-41fb-a6ec-750715335523\"},{\"content\":{\"connectorIds\":[\"Out1\",\"Out2\",\"Out3\",\"Out4\",\"Out5\"],\"side\":\"RIGHT\"},\"type\":\"ConnectorPlacement.EquallySpacedRectSide\",\"uuid\":\"d3309230-0110-441f-b944-3d5d4312a42e\"},{\"content\":{\"connectorIds\":[\"In6\"],\"side\":\"TOP\"},\"type\":\"ConnectorPlacement.EquallySpacedRectSide\",\"uuid\":\"012603a1-4678-4ae1-91f6-3e17a1c8130b\"}]},\"type\":\"ConnectorPlacement.EquallySpacedConnector\",\"uuid\":\"299866d5-057c-44fe-b725-733ff7b8fc12\"}],\"packageUris\":[\"http://schema.mathworks.com/mf0/Connector/19700101\"],\"version\":\"1.0\"}"
  iqd+-ref : Outport
  m : Outport  Port=2
  wires:
  Outer-loop/4(id-*) -> Mux/4
  Outer-loop/1(iq+*) -> Mux/1
  Outer-loop/3(iq-*) -> Mux/3
  Mux/1 -> iqd+-ref/1
  Qset/1 -> Outer-loop/2(Qset)
  Outer-loop/5(m) -> m/1
  Pset/1 -> Outer-loop/1(Pset)
  Outer-loop/2(id+*) -> Mux/2
  iqd+-/1 -> Outer-loop/4(iqd+-)
  freq/1 -> Outer-loop/5(freq)
  vqd+-/1 -> Outer-loop/3(vqd+-)
  Block/1 -> Outer-loop/6(Blk)

== system Scenario_1/G2/VSC/VSC Control/Control loops/Phasor PQ 1st ==
  Pset : Inport
  Qset : Inport  Port=2
  vqd+- : Inport  Port=3
  iqd+- : Inport  Port=4
  freq : Inport  Port=5
  Block : Inport  Port=6
  Mux : Mux
  Outer-loop : Subsystem
      settings: PortSchema="{\"entries\":[{\"content\":{\"sides\":[{\"content\":{\"connectorIds\":[\"In1\",\"In2\",\"In3\",\"In4\",\"In5\"]},\"type\":\"ConnectorPlacement.EquallySpacedRectSide\",\"uuid\":\"9a334ab0-c6a2-41fb-a6ec-750715335523\"},{\"content\":{\"connectorIds\":[\"Out1\",\"Out2\",\"Out3\",\"Out4\",\"Out5\"],\"side\":\"RIGHT\"},\"type\":\"ConnectorPlacement.EquallySpacedRectSide\",\"uuid\":\"d3309230-0110-441f-b944-3d5d4312a42e\"},{\"content\":{\"connectorIds\":[\"In6\"],\"side\":\"TOP\"},\"type\":\"ConnectorPlacement.EquallySpacedRectSide\",\"uuid\":\"012603a1-4678-4ae1-91f6-3e17a1c8130b\"}]},\"type\":\"ConnectorPlacement.EquallySpacedConnector\",\"uuid\":\"299866d5-057c-44fe-b725-733ff7b8fc12\"}],\"packageUris\":[\"http://schema.mathworks.com/mf0/Connector/19700101\"],\"version\":\"1.0\"}"
  iqd+-ref : Outport
  m : Outport  Port=2
  wires:
  Block/1 -> Outer-loop/6(Blk)
  vqd+-/1 -> Outer-loop/3(vqd+-)
  freq/1 -> Outer-loop/5(freq)
  iqd+-/1 -> Outer-loop/4(iqd+-)
  Outer-loop/2(id+*) -> Mux/2
  Pset/1 -> Outer-loop/1(Pset)
  Outer-loop/5(m) -> m/1
  Qset/1 -> Outer-loop/2(Qset)
  Mux/1 -> iqd+-ref/1
  Outer-loop/3(iq-*) -> Mux/3
  Outer-loop/1(iq+*) -> Mux/1
  Outer-loop/4(id-*) -> Mux/4

== system Scenario_1/G2/VSC/VSC Control/Control loops/SW, EMT AVG, Phasor Quasi-EMT ==
  Pset : Inport
  Qset : Inport  Port=2
  vqd+- : Inport  Port=3
  iqd+- : Inport  Port=4
  freq : Inport  Port=5
  Block : Inport  Port=6
  Inner-loop : Subsystem
      settings: PortSchema="{\"entries\":[{\"content\":{\"sides\":[{\"content\":{\"connectorIds\":[\"In1\",\"In2\",\"In3\",\"In4\"]},\"type\":\"ConnectorPlacement.EquallySpacedRectSide\",\"uuid\":\"8a2e5096-891c-4956-8b6b-4b283c05b7bc\"},{\"content\":{\"connectorIds\":[\"Out1\",\"Out2\",\"Out3\",\"Out4\"],\"side\":\"RIGHT\"},\"type\":\"ConnectorPlacement.EquallySpacedRectSide\",\"uuid\":\"b7af4d2f-ce3f-4dc6-8323-535c80ee1784\"},{\"content\":{\"connectorIds\":[\"In5\",\"In6\",\"In7\"],\"side\":\"TOP\"},\"type\":\"ConnectorPlacement.EquallySpacedRectSide\",\"uuid\":\"1131cb27-465f-45b8-a6a1-03893285239a\"},{\"content\":{\"connectorIds\":[],\"side\":\"BOTTOM\"},\"type\":\"ConnectorPlacement.EquallySpacedRectSide\",\"uuid\":\"c84e74f4-9dae-42a7-97b7-61f404019883\"}]},\"type\":\"ConnectorPlacement.EquallySpacedConnector\",\"uuid\":\"8a900364-1293-46a0-8824-7b0f85f5a81c\"}],\"packageUris\":[\"http://schema.mathworks.com/mf0/Connector/19700101\"],\"version\":\"1.0\"}"
  Mux : Mux
  Outer-loop : Subsystem
      settings: PortSchema="{\"entries\":[{\"content\":{\"sides\":[{\"content\":{\"connectorIds\":[\"In1\",\"In2\",\"In3\",\"In4\",\"In5\"]},\"type\":\"ConnectorPlacement.EquallySpacedRectSide\",\"uuid\":\"9a334ab0-c6a2-41fb-a6ec-750715335523\"},{\"content\":{\"connectorIds\":[\"Out1\",\"Out2\",\"Out3\",\"Out4\",\"Out5\"],\"side\":\"RIGHT\"},\"type\":\"ConnectorPlacement.EquallySpacedRectSide\",\"uuid\":\"d3309230-0110-441f-b944-3d5d4312a42e\"},{\"content\":{\"connectorIds\":[\"In6\"],\"side\":\"TOP\"},\"type\":\"ConnectorPlacement.EquallySpacedRectSide\",\"uuid\":\"012603a1-4678-4ae1-91f6-3e17a1c8130b\"}]},\"type\":\"ConnectorPlacement.EquallySpacedConnector\",\"uuid\":\"299866d5-057c-44fe-b725-733ff7b8fc12\"}],\"packageUris\":[\"http://schema.mathworks.com/mf0/Connector/19700101\"],\"version\":\"1.0\"}"
  vqd+-ref : Outport
  m : Outport  Port=2
  wires:
  Mux/1 -> vqd+-ref/1
  Inner-loop/4(vd-*) -> Mux/4
  Inner-loop/3(vq-*) -> Mux/3
  Inner-loop/2(vd+*) -> Mux/2
  Inner-loop/1(vq+*) -> Mux/1
  Outer-loop/4(id-*) -> Inner-loop/4(id-*)
  Pset/1 -> Outer-loop/1(Pset)
  Qset/1 -> Outer-loop/2(Qset)
  Outer-loop/5(m) -> m/1
  Outer-loop/3(iq-*) -> Inner-loop/3(iq-*)
  freq/1 -> Outer-loop/5(freq)
  iqd+-/1 -> Inner-loop/7(iqd+-), Outer-loop/4(iqd+-)
  Block/1 -> Inner-loop/5(Blk), Outer-loop/6(Blk)
  vqd+-/1 -> Inner-loop/6(vqd+-), Outer-loop/3(vqd+-)
  Outer-loop/2(id+*) -> Inner-loop/2(id+*)
  Outer-loop/1(iq+*) -> Inner-loop/1(iq+*)

== system Scenario_1/G2/VSC/VSC Control/Measurements/EMT ==
  note: abc to dq transformation
  Vabc : Inport
  Iabc : Inport  Port=2
  Gain2 : Gain  Gain=Vmv/Vhv
  Gain3 : Gain  Gain=Vhv/Vmv
  Iabc filter : powerlib_meascontrol/Filters/First-Order Filter  Commented=through  FilterType=Lowpass  Tc=tfilt  Ts=0  Initialize=off  Vac_Init=[0, 0, 60]  Vdc_Init=0  PlotResponse=off  FreqRange="[0,  200,  1]"
  Mux : Mux
  Mux2 : Mux
  Mux3 : Mux  Inputs=2
  PLL aligned with positive-sequence : Subsystem
  Phase-sequence separation2 : Subsystem
  Phase-sequence separation3 : Subsystem
  "Power (3ph, Instantaneous)" : powerlib_meascontrol/Measurements/Power (3ph, Instantaneous)
  Vabc filter : powerlib_meascontrol/Filters/First-Order Filter  Commented=through  FilterType=Lowpass  Tc=tfilt  Ts=0  Initialize=off  Vac_Init=[0, 0, 60]  Vdc_Init=0  PlotResponse=off  FreqRange="[0,  200,  1]"
  freq : Outport
  theta : Outport  Port=2
  vqd+- : Outport  Port=3
  iqd+- : Outport  Port=4
  PQabc : Outport  Port=5
  wires:
  Phase-sequence separation2/2(d+) -> Mux/2
  Phase-sequence separation2/1(q+) -> Mux/1
  Iabc filter/1 -> Gain3/1
  Gain2/1 -> PLL aligned with positive-sequence/1(Vabc), Phase-sequence separation2/1(abc)
  Gain3/1 -> Phase-sequence separation3/1(abc)
  PLL aligned with positive-sequence/1(theta) -> Phase-sequence separation3/2(Theta), theta/1, Phase-sequence separation2/2(Theta)  "theta"
  PLL aligned with positive-sequence/2(f) -> freq/1
  Iabc/1 -> Iabc filter/1, [Iabc]
  Vabc filter/1 -> Gain2/1
  Vabc/1 -> Vabc filter/1, [Vabc]
  Mux/1 -> vqd+-/1  "vqd+-"
  Mux2/1 -> iqd+-/1  "iqd+-"
  Phase-sequence separation2/3(q-) -> Mux/3
  Phase-sequence separation2/4(d-) -> Mux/4
  Phase-sequence separation3/1(q+) -> Mux2/1
  Phase-sequence separation3/2(d+) -> Mux2/2
  Phase-sequence separation3/3(q-) -> Mux2/3
  Phase-sequence separation3/4(d-) -> Mux2/4
  "Power (3ph, Instantaneous)"/2 -> Mux3/2
  "Power (3ph, Instantaneous)"/1 -> Mux3/1
  Mux3/1 -> PQabc/1  "PQ1"
  [Iabc] -> "Power (3ph, Instantaneous)"/2
  [Vabc] -> "Power (3ph, Instantaneous)"/1

== system Scenario_1/G2/VSC/VSC Control/Measurements/Phasor ==
  note: abc to dq transformation
      | (Phasor)
  Vabc : Inport
  Iabc : Inport  Port=2
  Complex to Magnitude-Angle : ComplexToMagnitudeAngle  Output=Angle
  Complex to Real-Imag{,1..3} (4 alike) : ComplexToRealImag
  Demux1 : Demux  Outputs=3
  Demux2 : Demux  Outputs=3
  Exp : Math  OutputSignalType=complex  SaturateOnIntegerOverflow=on
  Frequency (Phasor)1 : Subsystem  mask{f0=fg, Ts=5e-3}
      mask prompts: f0 "Fundamental frequency (Hz)"; Ts "Derivative filter time constant (s)"
  Gain{,3..4,6..7} (5 alike) : Gain  Gain=-1
  Gain1 : Gain  Gain=Vhv/Vmv
  Gain2 : Gain  Gain=Vmv/Vhv
  Gain5 : Gain  Gain=-1i
  Instantaneous power (Phasor) : Subsystem
  Mux1 : Mux
  Mux2 : Mux
  Mux3 : Mux  Inputs=2
  Product{1..4} (4 alike) : Product
  Subsystem : Subsystem
      mask init:
      | a = exp(1i*2*pi/3);
      | a2 = exp(1i*4*pi/3);
  Subsystem1 : Subsystem
      mask init:
      | a = exp(1i*2*pi/3);
      | a2 = exp(1i*4*pi/3);
  Subsystem3 : Subsystem
      mask init:
      | a = exp(1i*2*pi/3);
      | a2 = exp(1i*4*pi/3);
  Terminator2 : Terminator
  Terminator4 : Terminator
  vqd+- : Outport
  iqd+- : Outport  Port=2
  freq : Outport  Port=3
  theta : Outport  Port=4
  PQabc : Outport  Port=5
  wires:
  Gain7/1 -> Mux2/4
  Gain6/1 -> Mux2/3
  Exp/1 -> Product1/1, Product4/1, Product2/2, Product3/2
  Product3/1 -> Complex to Real-Imag/1
  Demux2/2 -> Product3/1
  Demux2/3 -> Product2/1
  Gain5/1 -> Exp/1
  Complex to Magnitude-Angle/1 -> Frequency (Phasor)1/1(Phase), Gain5/1, theta/1  "theta"
  Product4/1 -> Complex to Real-Imag1/1
  Complex to Real-Imag/2 -> Mux1/2  "vd+"
  Demux1/3 -> Product1/2
  Demux1/2 -> Product4/2
  Subsystem/1(012) -> Demux2/1
  Demux2/1 -> Terminator2/1
  Demux1/1 -> Terminator4/1
  Subsystem1/1(012) -> Demux1/1
  Subsystem3/1(seq+) -> Complex to Magnitude-Angle/1
  Frequency (Phasor)1/1(Freq) -> freq/1
  Vabc/1 -> [Vabc], Gain2/1
  Gain2/1 -> Subsystem3/1(abc), Subsystem/1(abc)
  Product2/1 -> Complex to Real-Imag2/1
  Product1/1 -> Complex to Real-Imag3/1
  Mux1/1 -> vqd+-/1
  Complex to Real-Imag/1 -> Mux1/1  "vq+"
  Complex to Real-Imag2/1 -> Gain/1  "vq-"
  Complex to Real-Imag2/2 -> Gain3/1  "vd-"
  Complex to Real-Imag1/1 -> Mux2/1  "iq+"
  Complex to Real-Imag1/2 -> Gain4/1  "id+"
  Complex to Real-Imag3/1 -> Gain6/1  "iq-"
  Complex to Real-Imag3/2 -> Gain7/1  "id-"
  Mux2/1 -> iqd+-/1
  Iabc/1 -> [Iabc], Gain1/1
  Gain1/1 -> Subsystem1/1(abc)
  Gain/1 -> Mux1/3
  Gain3/1 -> Mux1/4
  Gain4/1 -> Mux2/2
  [Iabc] -> Instantaneous power (Phasor)/2(Iabc)
  Instantaneous power (Phasor)/2(Q) -> Mux3/2
  Instantaneous power (Phasor)/1(P) -> Mux3/1
  [Vabc] -> Instantaneous power (Phasor)/1(Vabc)
  Mux3/1 -> PQabc/1

== system Scenario_1/G2/VSC/VSC Control/Modulation/EMT AVG ==
  note: Positive-sequence dq to abc
  note: Vref
  note: dq to abc
      | (AVG Model)
  note: negative-sequence dq to abc
  vqd+-* : Inport
  theta : Inport  Port=2
  Cartesian to Polar : simulink_extras/Transformations/Cartesian to Polar
  Cartesian to Polar1 : simulink_extras/Transformations/Cartesian to Polar
  Constant1 : Constant  Value=0
  Constant2 : Constant  Value=0
  Corrects delay : Subsystem
  Corrects delay1 : Subsystem
  Demux : Demux
  Gain : Gain  Gain=-1
  Gain2 : Gain  Gain=negseq_en
  Inverse Park Transform : eeTransforms/Inverse Park Transform  AxisAlignment=D-axis  PowerInvariant=off
  Inverse Park Transform1 : eeTransforms/Inverse Park Transform  AxisAlignment=D-axis  PowerInvariant=off
  Mux1 : Mux  Inputs=3
  Mux2 : Mux  Inputs=3
  Polar to Cartesian : simulink_extras/Transformations/Polar to Cartesian
      settings: SourceProductBaseCode=SL
  Polar to Cartesian1 : simulink_extras/Transformations/Polar to Cartesian
      settings: SourceProductBaseCode=SL
  Sum : Sum
  Sum1 : Sum  Inputs=|++
  Sum4 : Sum  Inputs=|++
  Unit Delay : UnitDelay  SampleTime=-1  HasFrameUpgradeWarning=on
  Ref : Outport
  wires:
  Demux/3 -> [vqnref]
  Demux/1 -> [vqpref]
  Demux/4 -> [vdnref]
  Demux/2 -> [vdpref]
  vqd+-*/1 -> Demux/1
  Gain2/1 -> Sum/2
  Polar to Cartesian/2 -> Mux1/2
  Sum4/1 -> Polar to Cartesian/2
  Mux1/1 -> Inverse Park Transform/1
  Cartesian to Polar/1 -> Polar to Cartesian/1
  [vdpref] -> Cartesian to Polar/1
  Cartesian to Polar/2 -> Sum4/1
  Constant1/1 -> Mux1/3
  [vqpref] -> Cartesian to Polar/2
  Corrects delay/1(dphi) -> Sum4/2
  Polar to Cartesian/1 -> Mux1/1
  Unit Delay/1 -> Ref/1
  [vdnref] -> Cartesian to Polar1/1
  Mux2/1 -> Inverse Park Transform1/1
  Cartesian to Polar1/1 -> Polar to Cartesian1/1
  Constant2/1 -> Mux2/3
  Polar to Cartesian1/2 -> Mux2/2
  Sum1/1 -> Polar to Cartesian1/2
  [vqnref] -> Cartesian to Polar1/2
  Corrects delay1/1(dphi) -> Sum1/2
  Gain/1 -> Inverse Park Transform1/2
  Polar to Cartesian1/1 -> Mux2/1
  Cartesian to Polar1/2 -> Sum1/1
  theta/1 -> Gain/1, Inverse Park Transform/2
  Sum/1 -> Unit Delay/1
  Inverse Park Transform/1 -> Sum/1
  Inverse Park Transform1/1 -> Gain2/1
